simulink model "ex8"  (R2019b)
settings: Solver=FixedStepAuto  StartTime=0.0  StopTime=Inf  FixedStep=FIXED_STEP_SIZE  RelTol=1e-3
values from neighbouring files (symbols this model uses):
  GAZEBO_SYNC_DT = 0.01    [position_interface_main.m]
  route = flip(route)    [astar_3d.m]    (also in maze_plotting_script.m = [1 1 1; 2 1 2; 3 1 3; 4 1 3; 5 1 3; 6 1 3]; position_interface_main.m = astar_3d(map, start, end_, 1))
undefined symbols (not defined in the file or in its folder): Angular, Linear
libraries: robotlib x4, robotgazebolib x1
settings Model: SimulationMode=external  Creator=ananda  LastModifiedBy=ubuntu
settings OptimizationCC: EnhancedBackFolding=on  PassReuseOutputArgsAs=Individual arguments  ZeroExternalMemoryAtStartup=off  ZeroInternalMemoryAtStartup=off  MaxStackSize=64  OptimizeBlockOrder=speed  DifferentSizesBufferReuse=on  OptimizationCustomize=off  EfficientTunableParamExpr=on
settings DebuggingCC: ParameterTunabilityLossMsg=error
settings HardwareCC: ProdBitPerPointer=32  ProdBitPerSizeT=32  ProdBitPerPtrDiffT=32  ProdLargestAtomicFloat=None  ProdIntDivRoundTo=Undefined  ProdEndianess=Unspecified  ProdWordSize=32  ProdHWDeviceType=Generic->Unspecified (assume 32-bit Generic)  UseEmbeddedCoderFeatures=off
settings SFSimCC: MATLABDynamicMemAlloc=off
settings RTWCC: SystemTargetFile=ert.tlc  HardwareBoard=Robot Operating System (ROS)  TLCOptions="-aInlineSetEventsForThisBaseRateFcn=TLC_FALSE -aSuppressMultiTaskScheduler=TLC_FALSE  -aRateBasedStepFcn=0"  TemplateMakefile=ert_default_tmf  GenerateReport=on  Toolchain=Catkin  IncludeHyperlinkInReport=on  LaunchReport=on  TargetLang=C++  GenerateTraceInfo=on  GenerateTraceReport=on  GenerateTraceReportSl=on  GenerateTraceReportSf=on  GenerateTraceReportEml=on
settings CodeAppCC: ForceParamTrailComments=on  IgnoreCustomStorageClasses=off  OperatorAnnotations=on  SimulinkDataObjDesc=on  SFDataObjDesc=on  InsertBlockDesc=on
settings ERTTargetCC: SupportNonInlinedSFcns=on

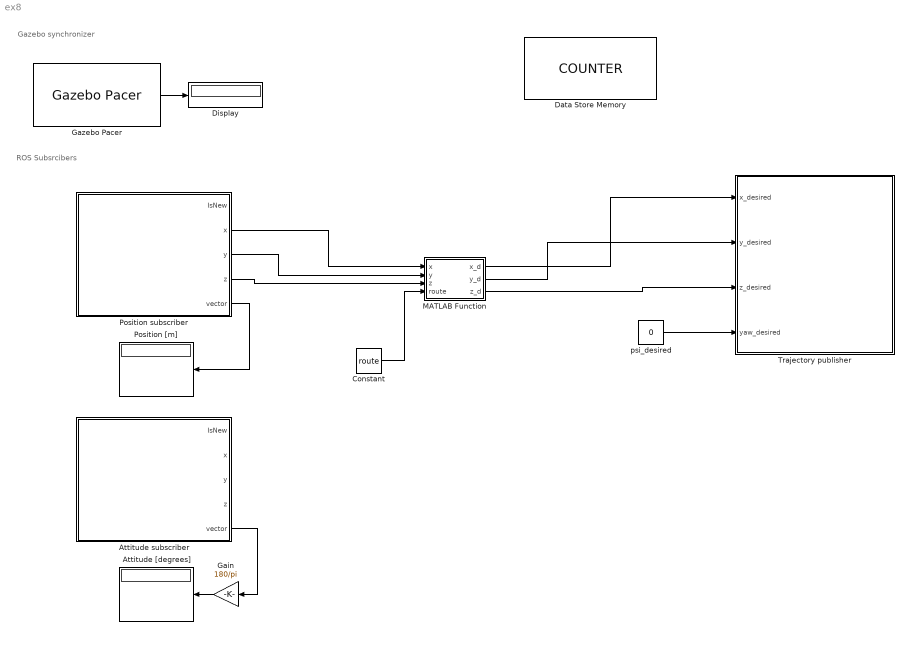
== system ex8 ==
  note: Gazebo synchronizer
  note: ROS Subsrcibers
  Attitude [degrees] : Display
  Attitude subscriber : Subsystem
  Constant : Constant  Value=route
  Data Store Memory : DataStoreMemory  DataStoreName=COUNTER  ReadBeforeWriteMsg=warning  WriteAfterWriteMsg=warning  WriteAfterReadMsg=warning  InitialValue=1  ShowAdditionalParam=off  OutDataTypeStr=double
  Display : Display
  Gain : Gain  Gain=180/pi
  Gazebo Pacer : robotgazebolib/Gazebo Pacer  ResetBehavior=Reset Gazebo simulation time  SampleTime=GAZEBO_SYNC_DT
      settings: SourceProductName=Robotics System Toolbox  SourceProductBaseCode=RO
  MATLAB Function : MATLAB Function  TreatAsAtomicUnit=on
  Position [m] : Display
  Position subscriber : Subsystem
  Trajectory publisher : Subsystem
  psi_desired : Constant  Value=0
  wires:
  Position subscriber/5(vector) -> Position [m]/1
  Attitude subscriber/5(vector) -> Gain/1
  Gain/1 -> Attitude [degrees]/1
  Gazebo Pacer/1 -> Display/1
  psi_desired/1 -> Trajectory publisher/4(yaw_desired)
  MATLAB Function/1(x_d) -> Trajectory publisher/1(x_desired)
  MATLAB Function/2(y_d) -> Trajectory publisher/2(y_desired)
  MATLAB Function/3(z_d) -> Trajectory publisher/3(z_desired)
  Position subscriber/2(x) -> MATLAB Function/1(x)
  Position subscriber/3(y) -> MATLAB Function/2(y)
  Position subscriber/4(z) -> MATLAB Function/3(z)
  Constant/1 -> MATLAB Function/4(route)

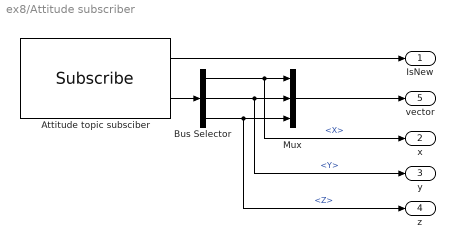
== system ex8/Attitude subscriber ==
  Attitude topic subsciber : robotlib/Subscribe  topicSource=Specify your own  topic=/hummingbird/orientation_rpy  messageType=geometry_msgs/Vector3  sampleTime=ATTI_SUB_DT  messageQueueLength=1
      settings: SourceProductName=ROS Toolbox
  Bus Selector : BusSelector  OutputSignals=X,Y,Z
  Mux : Mux  Inputs=3
  IsNew : Outport
  x : Outport  Port=2
  y : Outport  Port=3
  z : Outport  Port=4
  vector : Outport  Port=5
  wires:
  Bus Selector/3 -> z/1, Mux/3  "<Z>"
  Bus Selector/2 -> y/1, Mux/2  "<Y>"
  Bus Selector/1 -> x/1, Mux/1  "<X>"
  Attitude topic subsciber/2 -> Bus Selector/1
  Attitude topic subsciber/1 -> IsNew/1
  Mux/1 -> vector/1

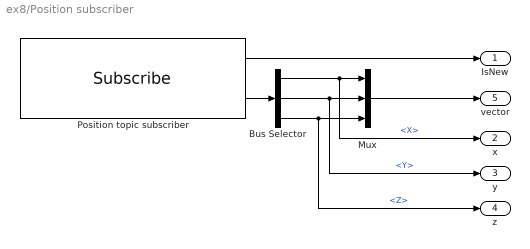
== system ex8/Position subscriber ==
  Bus Selector : BusSelector  OutputSignals=Point.X,Point.Y,Point.Z
  Mux : Mux  Inputs=3
  Position topic subscriber : robotlib/Subscribe  topicSource=Specify your own  topic=/hummingbird/odometry_sensor1/position  messageType=geometry_msgs/PointStamped  sampleTime=POS_SUB_DT  messageQueueLength=1
      settings: SourceProductName=ROS Toolbox
  IsNew : Outport
  x : Outport  Port=2
  y : Outport  Port=3
  z : Outport  Port=4
  vector : Outport  Port=5
  wires:
  Bus Selector/3 -> z/1, Mux/3  "<Z>"
  Bus Selector/2 -> y/1, Mux/2  "<Y>"
  Mux/1 -> vector/1
  Bus Selector/1 -> x/1, Mux/1  "<X>"
  Position topic subscriber/2 -> Bus Selector/1
  Position topic subscriber/1 -> IsNew/1

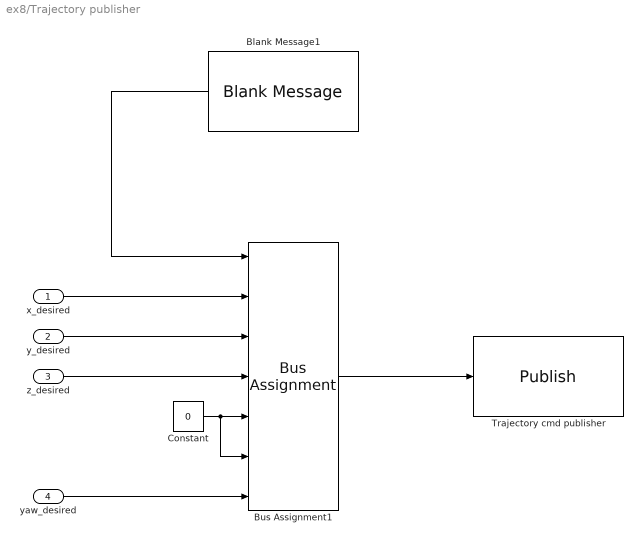
== system ex8/Trajectory publisher ==
  x_desired : Inport
  y_desired : Inport  Port=2
  z_desired : Inport  Port=3
  yaw_desired : Inport  Port=4
  Blank Message1 : robotlib/Blank Message  messageClass=Message  entityType=geometry_msgs/Twist  messageType=geometry_msgs/Twist  SampleTime=inf
      settings: SourceProductName=ROS Toolbox
  Bus Assignment1 : BusAssignment  AssignedSignals=Linear.X,Linear.Y,Linear.Z,Angular.X,Angular.Y,Angular.Z
  Constant : Constant  Value=0
  Trajectory cmd publisher : robotlib/Publish  topicSource=Specify your own  topic=/matlab/tracejtoryTwist  messageType=geometry_msgs/Twist  messageQueueLength=1
      settings: SourceProductName=ROS Toolbox
  wires:
  Blank Message1/1 -> Bus Assignment1/1
  Constant/1 -> Bus Assignment1/6, Bus Assignment1/5
  Bus Assignment1/1 -> Trajectory cmd publisher/1
  x_desired/1 -> Bus Assignment1/2
  y_desired/1 -> Bus Assignment1/3
  z_desired/1 -> Bus Assignment1/4
  yaw_desired/1 -> Bus Assignment1/7

== matlab function ex8/MATLAB Function ==
  data: x_d output; y_d output; z_d output; x input; y input; z input; COUNTER data_store_memory; route input
function [x_d,y_d,z_d] = fcn(x, y, z, route)
global COUNTER;
x_d = 0;
y_d = 0;
z_d = 0;
u = [x,y,z];
if isempty(u)
    u = [0,0,0];
    COUNTER = 1;
end
dist = norm(route(COUNTER, :)-u);
disp(route(COUNTER, :));
if dist<=0.1
    COUNTER = COUNTER+1;
end
if COUNTER>=size(route,1)
    COUNTER = size(route, 1);
end
x_d = route(COUNTER, 1);
y_d = route(COUNTER, 2);
z_d = route(COUNTER, 3);
end
